simulink model "fss2016a_"  (R2016a)
settings: Solver=FixedStepAuto  SolverMode=SingleTasking  StartTime=0.0  StopTime=t(end)  FixedStep=dt  RelTol=1e-3
values from neighbouring files (symbols this model uses):
  Ab = -a_0*T*eye(3)    [input_output.m]
  Asd = sysd.A    [input_output.m]
  Bb = T*eye(3)    [input_output.m]
  Bsd = sysd.B    [input_output.m]
  Cb = (b_0-a_0*b_1)*H    [input_output.m]
  Csd = sysd.C    [input_output.m]
  Db = b_1*H    [input_output.m]
  Dsd = sysd.D    [input_output.m]
  dt = 0.005    [input_output.m]
  GL = zeros(1,Nt-1);GL(1)=-alpha    [input_output.m]
  Reduce = zeros(3,54);Reduce(:,49:51)=eye(3)    [input_output.m]
  UL = i-1    [input_output.m]
  xb_initial = zeros(3,1)    [input_output.m]
  xs_initial = zeros(54,1)    [input_output.m]
settings Model: Creator=tujia  LastModifiedBy=li2920
settings DebuggingCC: SFUnexpectedBacktrackingDiag=error  SFNoUnconditionalDefaultTransitionDiag=error
settings GRTTargetCC: TargetLangStandard=C99 (ISO)  GeneratePreprocessorConditionals=Use local settings
settings ConfigComp: CovMetricSettings=dwe  CovHtmlReporting=off  CovSaveCumulativeToWorkspaceVar=off  CovSaveSingleToWorkspaceVar=off  CovExternalEMLEnable=on

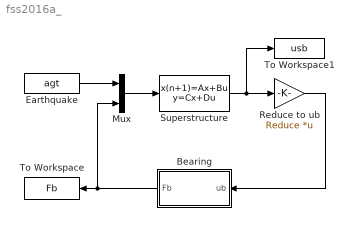
== system fss2016a_ ==
  Bearing : Subsystem
  Earthquake : FromWorkspace  VariableName=agt  SampleTime=0
  Mux : Mux  Inputs=2
  Reduce to ub : Gain  Gain=Reduce  Multiplication=Matrix(K*u)
  Superstructure : DiscreteStateSpace  A=Asd  B=Bsd  C=Csd  D=Dsd  X0=xs_initial  SampleTime=dt
  To Workspace : ToWorkspace  VariableName=Fb  SaveFormat=Timeseries  SampleTime=dt
      settings: Save2DSignal=2-D array (concatenate along first dimension)
  To Workspace1 : ToWorkspace  VariableName=usb  SaveFormat=Timeseries  SampleTime=dt
      settings: Save2DSignal=2-D array (concatenate along first dimension)
  wires:
  Reduce to ub/1 -> Bearing/1(ub)
  Mux/1 -> Superstructure/1
  Superstructure/1 -> Reduce to ub/1, To Workspace1/1
  Earthquake/1 -> Mux/1
  Bearing/1(Fb) -> Mux/2, To Workspace/1

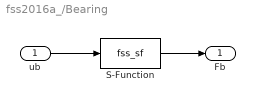
== system fss2016a_/Bearing ==
  ub : Inport
  S-Function : S-Function  FunctionName=fss_sf  Parameters=UL,GL,Ab,Bb,Cb,Db,xb_initial  SFunctionDeploymentMode=off  EnableBusSupport=off
  Fb : Outport
  wires:
  ub/1 -> S-Function/1
  S-Function/1 -> Fb/1
